simulink model "lab08a"  (Simulink 5.0)
settings: Solver=ode45  StartTime=0.0  StopTime=10.0  RelTol=1e-3
settings Model: LastModifiedBy=Frank Gloria

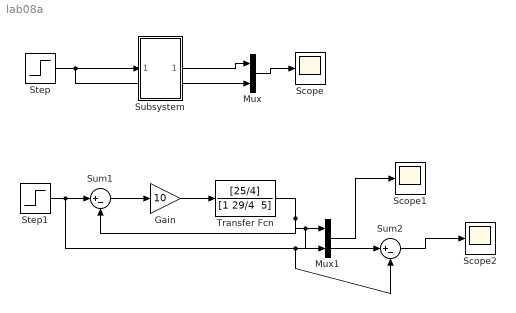
== system lab08a ==
  Gain : Gain  Gain=10  SaturateOnIntegerOverflow=on
  Mux : Mux  Inputs=2
  Mux1 : Mux  Inputs=2
  Scope : Scope
  Scope1 : Scope
  Scope2 : Scope
      settings: SaveName=ScopeData2
  Step : Step  Time=0  Before=1  SampleTime=0
  Step1 : Step  Time=0  Before=1  SampleTime=0
  Subsystem : Subsystem  mask{K=8}
      mask prompts: K "Ganho"
  Sum1 : Sum  Inputs=|+-  SaturateOnIntegerOverflow=on
  Sum2 : Sum  Inputs=|+-  SaturateOnIntegerOverflow=on
  Transfer Fcn : TransferFcn  Numerator=[25/4]  Denominator="[1 29/4  5]"
  wires:
  Step1/1 -> Sum1/1, Sum2/2, Mux1/2
  Sum1/1 -> Gain/1
  Gain/1 -> Transfer Fcn/1
  Step/1 -> Subsystem/1(In1), Mux/2
  Subsystem/1(Out1) -> Mux/1
  Mux/1 -> Scope/1
  Mux1/1 -> Scope1/1
  Transfer Fcn/1 -> Sum1/2, Mux1/1, Sum2/1
  Sum2/1 -> Scope2/1

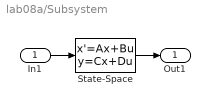
== system lab08a/Subsystem ==
  In1 : Inport
  State-Space : StateSpace  A=[-7.5 5+7.5*K; -1 K]  B=[-5; 0]  C=[0 1+K]  D=0
  Out1 : Outport
  wires:
  In1/1 -> State-Space/1
  State-Space/1 -> Out1/1
